simulink model "ExampleSimpleVehicle_PID"  (R2024b)
settings: Solver=ode1  StartTime=0.0  StopTime=inf  FixedStep=0.01  RelTol=1e-3
undefined symbols (not defined in the file or in its folder): DiscIntNeverNeededParam
libraries: rFproPhysicsLib x14, slpidlib x2, simulink x1
settings Model: ParamWorkspaceSource=ReferencedWorkspace  TunableVars=LOCAL_PORT_RECV,REMOTE_PORT_RECV,gCGHeight,gFrontTrack,gFrontWheelRadius,gLeftWheelBase,gRearTrack,gRearWheelRadius,gRightWheelBase  TunableVarsStorageClass=Auto,Auto,Auto,Auto,Auto,Auto,Auto,Auto,Auto  TunableVarsTypeQualifier=,,,,,,,,  Creator=enewton  LastModifiedBy=Saian
settings SolverCC: AlgebraicLoopSolver=TrustRegion
settings DataIOCC: LimitDataPoints=on  SaveFormat=Array  SignalLoggingSaveFormat=ModelDataLogs  SaveOutput=off  SignalLogging=off  DSMLogging=off  SaveTime=off  ReturnWorkspaceOutputs=off
settings OptimizationCC: BlockReduction=off  ConditionallyExecuteInputs=off  OptimizeBlockIOStorage=off  BufferReuse=off  GlobalBufferReuse=off  ExpressionFolding=off  ExpressionDepthLimit=2147483647  LocalBlockOutputs=off  LifeSpan=inf  OptimizeDataStoreBuffers=off  BusAssignmentInplaceUpdate=off
settings DebuggingCC: UnderspecifiedInitializationDetection=Classic  MergeDetectMultiDrivingBlocksExec=none  SolverPrmCheckMsg=warning  FcnCallInpInsideContextMsg=warning  UnconnectedInputMsg=warning  UnconnectedOutputMsg=warning  UnconnectedLineMsg=warning  StateNameClashWarn=warning  SFUnexpectedBacktrackingDiag=warning  SFNoUnconditionalDefaultTransitionDiag=warning  SFExecutionAtInitializationDiag=none  ArithmeticOperatorsInVariantConditions=warning
settings HardwareCC: ProdBitPerPointer=32  ProdBitPerSizeT=32  ProdBitPerPtrDiffT=32  ProdLargestAtomicFloat=None  ProdIntDivRoundTo=Undefined  ProdEndianess=Unspecified  ProdWordSize=32  ProdHWDeviceType=32-bit Generic
settings ModelReferenceCC: EnableRefExpFcnMdlSchedulingChecks=on  PropagateSignalLabelsOutOfModel=off
settings SFSimCC: SimUseLocalCustomCode=off  CustomCodeUndefinedFunction=UseInterfaceOnly  SimTargetLang=C++
settings RTWCC: Description=rFpro Target (Run Physics)  SystemTargetFile=rfpro.tlc  MakeCommand="make_rtw OPTS=\"-DRUN_PHYSICS\""  TemplateMakefile=rfpro.tmf  RTWUseLocalCustomCode=off  TargetLang=C++  GPUComputeCapability=3.5
settings CodeAppCC: StateflowObjectComments=on
settings STFCustomTargetCC: ModelReferenceCompliant=off  CombineOutputUpdateFcns=on  MatFileLogging=on  CPPClassGenCompliant=on  SystemTargetFile=rfpro.tlc
settings GRTTargetCC: TargetLangStandard=C89/C90 (ANSI)  ModelReferenceCompliant=off  ParMdlRefBuildCompliant=off  CompOptLevelCompliant=off  ConcurrentExecutionCompliant=off  UseToolchainInfoCompliant=off
settings ConfigComp: CovMetricSettings=dw  CovSaveCumulativeToWorkspaceVar=on  CovSaveSingleToWorkspaceVar=on  CovExternalEMLEnable=off

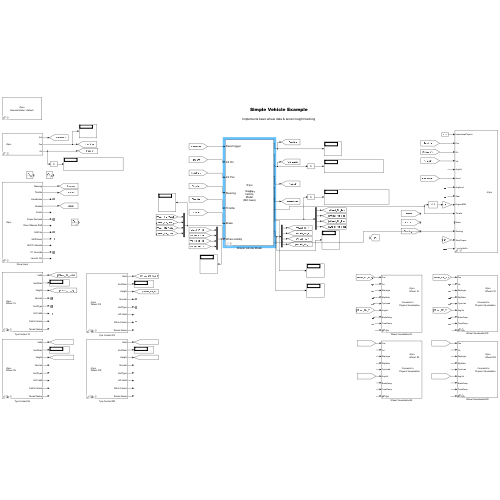
[thumbnail: Simulink's stored preview of the top-level diagram]
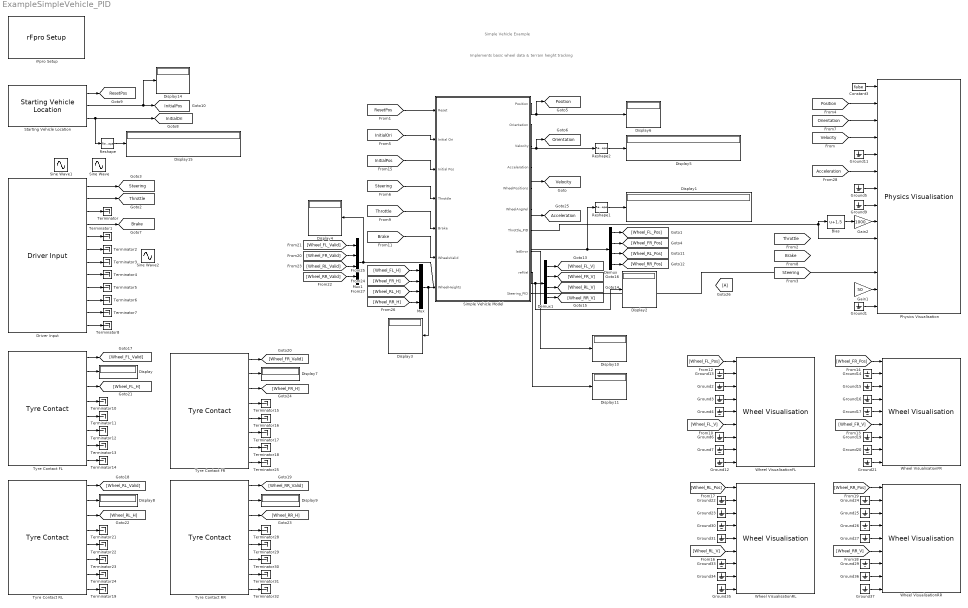
== system ExampleSimpleVehicle_PID ==
  note: Simple Vehicle Example
  note: Implements basic wheel data & terrain height tracking
  Bias : Bias  Bias=1.5  SaturateOnIntegerOverflow=off
  Constant3 : Constant  Value=false
  Demux : Demux
  Demux1 : Demux
  Display{,1..11,14..15} (14 alike) : Display
  "Driver Input " : rFproPhysicsLib/Driver Input
      settings: SourceProductName=rFpro Physics
  Gain1 : Gain  Gain=50
  Gain2 : Gain  Gain=1000
  Goto26 : Goto
  Ground{1..7,9,11..17,19..27,29..31,33..37} (32 alike) : Ground
  Mux : Mux
  Mux1 : Mux
  Physics Visualisation : rFproPhysicsLib/Physics Visualisation  PAR_SKIP_INTERNAL_PHYSICS=off  PAR_ACCEL_VALID=on  PAR_ROT_ACCEL_VALID=off  PAR_GEAR_VALID=off  PAR_RPM_VALID=on  PAR_INPUTS_VALID=on  PAR_STEER_TORQUE_VALID=on  PAR_HEADLIGHTS_ON_VALID=off  PAR_WHEEL_POS_VALID=on  PAR_WHEEL_ORI_VALID=off  PAR_TYRE_PARAMS_VALID=off  PAR_WHEEL_ROTATION_VALID=on  PAR_WHEEL_BRAKE_TEMP_VALID=off  PAR_WHEEL_TREAD_TEMP_VALID=off  PAR_WHEEL_AIR_TEMP_VALID=off  period=-1  offset=0  useReverseByteOrder=on  rFpro__platform=Remote Model - Default
      settings: SourceProductName=rFpro Physics
  Reshape : Reshape  OutputDimensionality=Customize  OutputDimensions=[3,3]
  Reshape1 : Reshape  OutputDimensionality=Customize  OutputDimensions=[3,4]
  Reshape2 : Reshape  OutputDimensionality=Customize  OutputDimensions=[3,3]
  Simple Vehicle Model : Subsystem  AncestorBlock=rFproPhysicsLib/Internal Utility/Simple Vehicle Model  mask(rFpro Simple Vehicle Model){TIMESTEP=0.01, gCGHeight=0.52, gLeftWheelBase=2.626, gRightWheelBase=2.626, gFrontTrack=1.55, gRearTrack=1.525, gFrontWheelRadius=0.32, gRearWheelRadius=0.33, gWheelDeflection=0}
      mask prompts: TIMESTEP "Sample time"; gCGHeight "Height of car body ref point"; gLeftWheelBase "Left Wheel Base"; gRightWheelBase "Right Wheel Base"; gFrontTrack "Front Wheel Track"; gRearTrack "Rear Wheel Track"; gFrontWheelRadius "Front wheel radius"; gRearWheelRadius "Rear wheel radius"; gWheelDeflection "Wheel Deflection"
      mask help:
      | Enter the car dimensions in metres.
      |
      | This block creates a CG_OFFSET_FROM_NOSE variable in the base workspace, for use by the "Starting Vehicle Location" block.
      mask init:
      | assignin('base', 'CG_OFFSET_FROM_NOSE', [-gLeftWheelBase/2, 0, gCGHeight]);
      mask DialogControl Container5 Prompt: Block Parameters
      mask DialogControl ParameterGroupVar Prompt: Vehicle Parameters
      mask Display:
      | disp('rFpro\n\nSimple\nVehicle\nModel\n(ISO Axes)')
      | port_label('input', 1, 'Reset trigger')
      | port_label('input', 2, 'Init Ori')
      | port_label('input', 3, 'Init Pos')
      | port_label('input', 4, 'Steering')
      | port_label('input', 5, 'Throttle')
      | port_label('input', 6, 'Brake')
      | port_label('input', 7, 'Wheel validity')
      | port_label('input', 8, 'Wheel heights')
      | 
      | port_label('output', 1, 'Position')
      | port_label('output', 2, 'Orientation')
      | port_label('output', 3, 'Velocity')
      | port_label('output', 4, 'Acceleration')
      | port_label('output', 5, 'Pos of Wheels')
      | port_label('output', 6, 'AngVel of Wheels')
  Sine Wave : Sin  SampleTime=0
  Sine Wave1 : Sin  Amplitude=0.5  Bias=0.5  Phase=pi  SampleTime=0
  Sine Wave2 : Sin  Amplitude=0.5  Bias=0.5  SampleTime=0
  Starting Vehicle Location : rFproPhysicsLib/Starting Vehicle Location  cg_offset=CG_OFFSET_FROM_NOSE  numPackets=1  rFpro__platform=Remote Model - Default
      settings: SourceProductName=rFpro Physics
  Terminator{,1..8,10..19,21..25,28..32} (29 alike) : Terminator
  Tyre Contact FL : rFproPhysicsLib/Tyre Contact  LabelModeActiveChoice=rFproLib_RemoteModel  wheel=FL  contact=[]  radius=0.3  width=0.32  sampleTime=0.001  rFpro__platform=Remote Model - Default
      settings: SourceProductName=rFpro Physics
  Tyre Contact FR : rFproPhysicsLib/Tyre Contact  LabelModeActiveChoice=rFproLib_RemoteModel  wheel=FR  contact=[]  radius=0.32  width=0.25  sampleTime=0.001  rFpro__platform=Remote Model - Default
      settings: SourceProductName=rFpro Physics
  Tyre Contact RL : rFproPhysicsLib/Tyre Contact  LabelModeActiveChoice=rFproLib_RemoteModel  wheel=RL  contact=[]  radius=0.33  width=0.25  sampleTime=0.001  rFpro__platform=Remote Model - Default
      settings: SourceProductName=rFpro Physics
  Tyre Contact RR : rFproPhysicsLib/Tyre Contact  LabelModeActiveChoice=rFproLib_RemoteModel  wheel=RR  contact=[]  radius=0.33  width=0.25  sampleTime=0.001  rFpro__platform=Remote Model - Default
      settings: SourceProductName=rFpro Physics
  Wheel VisualisationFL : rFproPhysicsLib/Wheel Visualisation  wheelStr=FL
      settings: SourceProductName=rFpro Physics
  Wheel VisualisationFR : rFproPhysicsLib/Wheel Visualisation  wheelStr=FR
      settings: SourceProductName=rFpro Physics
  Wheel VisualisationRL : rFproPhysicsLib/Wheel Visualisation  wheelStr=RL
      settings: SourceProductName=rFpro Physics
  Wheel VisualisationRR : rFproPhysicsLib/Wheel Visualisation  wheelStr=RR
      settings: SourceProductName=rFpro Physics
  rFpro Setup : rFproPhysicsLib/rFpro Setup  platform=Remote Model - Default  stopOnSessionEnd=on  usePseudoRealtime=on  syncToRF=on  useReverseByteOrder=off  useRfTime=on  minIterations=4  maxIterations=1000  ipReceiveAddress='127.0.0.1'  ipReceivePort=11054  receiveSampleTime=-1  ipTransmitAddress='127.0.0.1'  ipTransmitPort=11052  transmitSampleTime=-1  pluginType=RUN_PHYSICS  sysTarget=xpctarget.tlc  templateMakeFile=xpc_default_tmf  makeCommand=make_rtw  buildDesc=xPC target
      settings: SourceProductName=rFpro Physics
  tag scope: Acceleration=global, Brake=global, InitialOri=global, InitialPos=global, Orientation=global, Position=global, ResetPos=global, Steering=global, Throttle=global, Velocity=global
  wires:
  Starting Vehicle Location/2 -> Display14/1, [InitialPos]
  Constant3/1 -> Physics Visualisation/1
  [Orientation] -> Physics Visualisation/3
  [Velocity] -> Physics Visualisation/4
  [Position] -> Physics Visualisation/2
  "Driver Input "/3 -> Terminator/1
  "Driver Input "/5 -> Terminator1/1
  "Driver Input "/6 -> Terminator2/1
  "Driver Input "/7 -> Terminator3/1
  "Driver Input "/8 -> Terminator4/1
  "Driver Input "/9 -> Terminator5/1
  "Driver Input "/10 -> Terminator6/1
  "Driver Input "/11 -> Terminator7/1
  "Driver Input "/12 -> Terminator8/1
  [Acceleration] -> Physics Visualisation/6
  Ground9/1 -> Physics Visualisation/8
  Gain2/1 -> Physics Visualisation/9
  Ground11/1 -> Physics Visualisation/5
  Starting Vehicle Location/1 -> [ResetPos]
  Gain1/1 -> Physics Visualisation/13
  Ground1/1 -> Physics Visualisation/14
  Tyre Contact FL/4 -> Terminator10/1
  Tyre Contact FL/5 -> Terminator11/1
  Tyre Contact FL/6 -> Terminator12/1
  Ground2/1 -> Wheel VisualisationFL/3
  Ground3/1 -> Wheel VisualisationFL/4
  Ground4/1 -> Wheel VisualisationFL/5
  Ground6/1 -> Wheel VisualisationFL/7
  Ground7/1 -> Wheel VisualisationFL/8
  Ground12/1 -> Wheel VisualisationFL/9
  Ground13/1 -> Wheel VisualisationFL/2
  Tyre Contact FL/7 -> Terminator13/1
  Tyre Contact FL/2 -> Display/1
  Tyre Contact FL/8 -> Terminator14/1
  Tyre Contact FR/5 -> Terminator16/1
  Tyre Contact FR/6 -> Terminator17/1
  Tyre Contact FR/7 -> Terminator18/1
  Tyre Contact FR/2 -> Display7/1
  Tyre Contact RL/4 -> Terminator21/1
  Tyre Contact RL/5 -> Terminator22/1
  Tyre Contact RL/6 -> Terminator23/1
  Tyre Contact RL/7 -> Terminator24/1
  Tyre Contact RL/2 -> Display8/1
  Tyre Contact RL/8 -> Terminator19/1
  Tyre Contact RR/5 -> Terminator29/1
  Tyre Contact RR/6 -> Terminator30/1
  Tyre Contact RR/7 -> Terminator31/1
  Tyre Contact RR/2 -> Display9/1
  Ground14/1 -> Wheel VisualisationFR/2
  Ground15/1 -> Wheel VisualisationFR/3
  Ground16/1 -> Wheel VisualisationFR/4
  Ground17/1 -> Wheel VisualisationFR/5
  Ground19/1 -> Wheel VisualisationFR/7
  Ground20/1 -> Wheel VisualisationFR/8
  Ground21/1 -> Wheel VisualisationFR/9
  Ground22/1 -> Wheel VisualisationRL/2
  Ground23/1 -> Wheel VisualisationRL/3
  Ground30/1 -> Wheel VisualisationRL/4
  Ground31/1 -> Wheel VisualisationRL/5
  Ground33/1 -> Wheel VisualisationRL/7
  Ground34/1 -> Wheel VisualisationRL/8
  Ground35/1 -> Wheel VisualisationRL/9
  Ground24/1 -> Wheel VisualisationRR/2
  Ground25/1 -> Wheel VisualisationRR/3
  Ground26/1 -> Wheel VisualisationRR/4
  Ground27/1 -> Wheel VisualisationRR/5
  Ground29/1 -> Wheel VisualisationRR/7
  Ground36/1 -> Wheel VisualisationRR/8
  Ground37/1 -> Wheel VisualisationRR/9
  Ground5/1 -> Physics Visualisation/7
  Starting Vehicle Location/3 -> Reshape/1, [InitialOri]
  [InitialOri] -> Simple Vehicle Model/2(Initial Ori)
  [ResetPos] -> Simple Vehicle Model/1(Reset)
  [Throttle] -> Simple Vehicle Model/5(Brake)
  [Brake] -> Simple Vehicle Model/6(WheelsValid)
  [InitialPos] -> Simple Vehicle Model/3(Initial Pos)
  [Steering] -> Simple Vehicle Model/4(Throttle)
  Simple Vehicle Model/5(WheelPositions) -> Reshape1/1, Demux/1
  Tyre Contact FR/4 -> Terminator15/1
  Tyre Contact FR/8 -> Terminator25/1
  Simple Vehicle Model/1(Position) -> Display6/1, [Position]
  Simple Vehicle Model/2(Orientation) -> [Orientation], Reshape2/1
  Simple Vehicle Model/3(Velocity) -> [Velocity]
  Demux/1 -> [Wheel_FL_Pos]
  Demux/2 -> [Wheel_FR_Pos]
  Demux/3 -> [Wheel_RL_Pos]
  Demux/4 -> [Wheel_RR_Pos]
  Demux1/1 -> [Wheel_FL_V]
  Demux1/2 -> [Wheel_FR_V]
  Demux1/3 -> [Wheel_RL_V]
  Demux1/4 -> [Wheel_RR_V]
  Simple Vehicle Model/6(WheelAngVel) -> Display2/1, Demux1/1
  [Wheel_FL_Pos] -> Wheel VisualisationFL/1
  [Wheel_FL_V] -> Wheel VisualisationFL/6
  [Wheel_FR_Pos] -> Wheel VisualisationFR/1
  [Wheel_FR_V] -> Wheel VisualisationFR/6
  [Wheel_RL_V] -> Wheel VisualisationRL/6
  [Wheel_RL_Pos] -> Wheel VisualisationRL/1
  [Wheel_RR_V] -> Wheel VisualisationRR/6
  [Wheel_RR_Pos] -> Wheel VisualisationRR/1
  Tyre Contact RL/1 -> [Wheel_RL_Valid]
  Tyre Contact RL/3 -> [Wheel_RL_H]
  Tyre Contact RR/1 -> [Wheel_RR_Valid]
  Tyre Contact RR/3 -> [Wheel_RR_H]
  Tyre Contact FR/3 -> [Wheel_FR_H]
  Tyre Contact FR/1 -> [Wheel_FR_Valid]
  Tyre Contact FL/1 -> [Wheel_FL_Valid]
  Tyre Contact FL/3 -> [Wheel_FL_H]
  [Wheel_RL_Valid] -> Mux1/3
  [Wheel_RR_Valid] -> Mux1/4
  [Wheel_FL_Valid] -> Mux1/1
  [Wheel_FR_Valid] -> Mux1/2
  [Wheel_FR_H] -> Mux/2
  [Wheel_FL_H] -> Mux/1
  [Wheel_RR_H] -> Mux/4
  [Wheel_RL_H] -> Mux/3
  Mux1/1 -> Display4/1, Simple Vehicle Model/7(WheelHeights)
  Mux/1 -> Display3/1
  Tyre Contact RR/4 -> Terminator28/1
  Tyre Contact RR/8 -> Terminator32/1
  Reshape/1 -> Display15/1
  Reshape1/1 -> Display1/1
  Reshape2/1 -> Display5/1
  Bias/1 -> Gain2/1
  Simple Vehicle Model/4(Acceleration) -> [Acceleration]
  "Driver Input "/1 -> [Steering]
  "Driver Input "/2 -> [Throttle]
  "Driver Input "/4 -> [Brake]
  Simple Vehicle Model/8(latError) -> Display10/1
  Simple Vehicle Model/9(refVel) -> Display11/1
  Simple Vehicle Model/7(Throttle_PID) -> Bias/1, Physics Visualisation/10
  Simple Vehicle Model/10(Steering_PID) -> Physics Visualisation/12

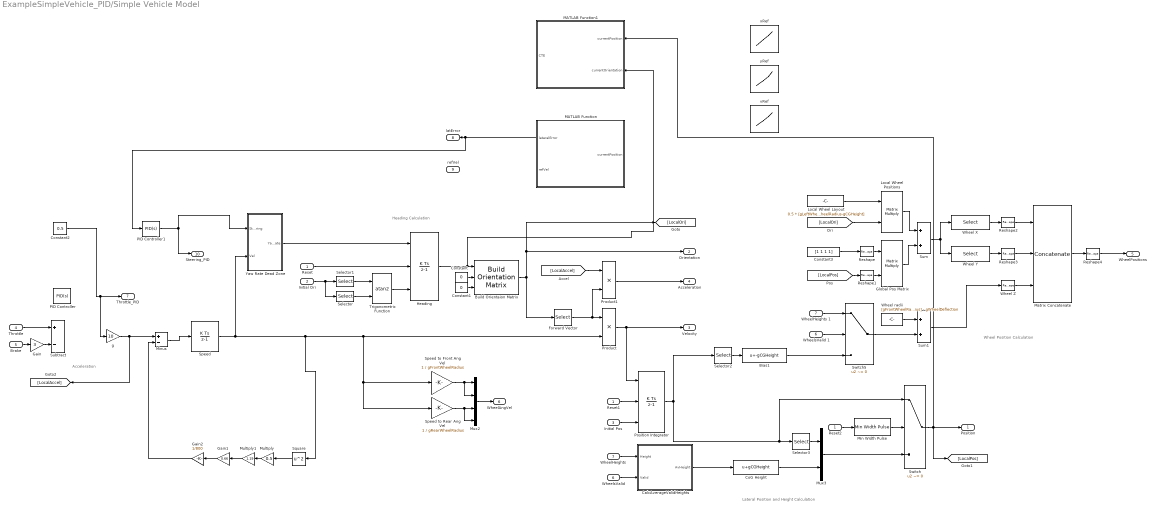
== system ExampleSimpleVehicle_PID/Simple Vehicle Model ==
  note: Wheel Position Calculation
  note: Acceleration
  note: Heading Calculation
  note: Lateral Position and Height Calculation
  Reset : Inport
  Initial Ori : Inport  Port=2
  Initial Pos : Inport  Port=3
  Throttle : Inport  Port=4
  Brake : Inport  Port=5
  WheelsValid : Inport  Port=6
  WheelHeights : Inport  Port=7
  Bias1 : Bias  Bias=-gCGHeight  SaturateOnIntegerOverflow=off
  Build Orientaion Matrix : rFproPhysicsLib/Build Orientation Matrix  ISOAxes=on  YPROrder=on
      settings: SourceProductName=rFpro Physics
  CalcAverageValidHeights : Subsystem
  CoG Height : Bias  Bias=gCGHeight  SaturateOnIntegerOverflow=off
  Constant : Constant  Value=0
  Constant1 : Constant  Value=0
  Constant2 : Constant  Value=0.5
  Constant3 : Constant  Value=[1 1 1 1]
  Forward Vector : Selector  NumberOfDimensions=2  InputPortWidth=3  IndexOptions=Index vector (dialog),Index vector (dialog)  Indices=1,1:3  OutputSizes=1,1
  Gain : Gain  Gain=3
  Gain1 : Gain  Gain=0.66
  Gain2 : Gain  Gain=1/800
  Global Pos Matrix : Product  Multiplication=Matrix(*)
  Heading : DiscreteIntegrator  ExternalReset=level  InitialConditionSource=external  SampleTime=TIMESTEP  ICPrevOutput=DiscIntNeverNeededParam  ICPrevScaledInput=DiscIntNeverNeededParam
  Local Wheel Positions : Product  Multiplication=Matrix(*)  RndMeth=Zero
  Local Wheel Layout : Constant  Value="0.5 * [gLeftWheelBase,   gFrontTrack, gFrontWheelRadius-gCGHeight; gRightWheelBase, -gFrontTrack, gFrontWheelRadius-gCGHeight; -gLeftWheelBase,   gRearTrack,  gRearWheelRadius-gCGHeight; -gRightWheelBase, -gRearTrack,  gRearWheelRadius-gCGHeight]"
  MATLAB Function : MATLAB Function  TreatAsAtomicUnit=on
  MATLAB Function1 : MATLAB Function  AncestorBlock=rFproPhysicsLib/Internal Utility/Simple Vehicle Model/MATLAB Function  TreatAsAtomicUnit=on
  Matrix Concatenate : Concatenate  NumInputs=3  Mode=Multidimensional array
  Min Width Pulse : rFproPhysicsLib/Internal Utility/Min Width Pulse  width=20
      settings: SourceProductName=rFpro Physics
  Minus : Sum  Inputs=+-
  Multiply : Gain  Gain=0.5
  Multiply1 : Gain  Gain=1.19
  Mux2 : Mux
  Mux3 : Mux  Inputs=2
  PID Controller : slpidlib/PID Controller  Controller=PID  Form=Parallel  TimeDomain=Continuous-time  UseExternalTs=off  SampleTime=-1  IntegratorMethod=Forward Euler  FilterMethod=Forward Euler  ControllerParametersSource=internal  P=1  I=0  UseKiTs=off  D=5  UseExternalDerivativeSource=off  N=100  UseFilter=on  TunerSelectOption=Transfer Function Based (PID Tuner App)  InitialConditionSource=internal  InitialConditionForIntegrator=0  InitialConditionForFilter=0  DifferentiatorICPrevScaledInput=0  ExternalReset=none  TrackingMode=off  Kt=1  LimitOutput=on  SatLimitsSource=internal  UpperSaturationLimit=1  LowerSaturationLimit=-1  LinearizeAsGain=on  AntiWindupMode=none  Kb=1  LimitIntegrator=off  UpperIntegratorSaturationLimit=inf  LowerIntegratorSaturationLimit=-inf  POutMin=[]  POutMax=[]  IOutMin=[]  IOutMax=[]  DOutMin=[]  DOutMax=[]  NOutMin=[]  NOutMax=[]  SumOutMin=[]  SumOutMax=[]  SaturationOutMin=[]  SaturationOutMax=[]  PParamMin=[]  PParamMax=[]  IParamMin=[]  IParamMax=[]  DParamMin=[]  DParamMax=[]  NParamMin=[]  NParamMax=[]  KbParamMin=[]  KbParamMax=[]  KtParamMin=[]  KtParamMax=[]  KbOutMin=[]  KbOutMax=[]  KtOutMin=[]  KtOutMax=[]  IntegratorOutMin=[]  IntegratorOutMax=[]  FilterOutMin=[]  FilterOutMax=[]  SumI1OutMin=[]  SumI1OutMax=[]  SumI2OutMin=[]  SumI2OutMax=[]  SumI3OutMin=[]  SumI3OutMax=[]  SumI4OutMin=[]  SumI4OutMax=[]  SumDOutMin=[]  SumDOutMax=[]  DifferentiatorOutMin=[]  DifferentiatorOutMax=[]  FilterDiffOutCoefMin=[]  FilterDiffOutCoefMax=[]  ReciprocalOutMin=[]  ReciprocalOutMax=[]  SumDenOutMin=[]  SumDenOutMax=[]  SumNumOutMin=[]  SumNumOutMax=[]  DivideOutMin=[]  DivideOutMax=[]  UdiffTsProdOutMin=[]  UdiffTsProdOutMax=[]  NTsProdOutMin=[]  NTsProdOutMax=[]  UintegralTsProdOutMin=[]  UintegralTsProdOutMax=[]  UngainTsProdOutMin=[]  UngainTsProdOutMax=[]  ClampingZeroOutDataTypeStr=Inherit: Inherit via back propagation  ClampingZeroOutMin=[]  ClampingZeroOutMax=[]  FilterDenConstantOutDataTypeStr=Inherit: Inherit via back propagation  FilterDenConstantOutMin=[]  FilterDenConstantOutMax=[]  PCopyOutDataTypeStr=Inherit: Inherit via back propagation  PCopyOutMin=[]  PCopyOutMax=[]  NCopyOutDataTypeStr=Inherit: Inherit via back propagation  NCopyOutMin=[]  NCopyOutMax=[]  IntegratorContinuousStateAttributes=''  IntegratorStateMustResolveToSignalObject=off  IntegratorRTWStateStorageClass=Auto  FilterContinuousStateAttributes=''  FilterStateMustResolveToSignalObject=off  FilterRTWStateStorageClass=Auto  ParallelPVariant=InternalParameters  IdealPVariant=Disabled  IVariant=InternalParameters  DVariant=InternalParameters  IntegratorVariant=Continuous  SatVariant=Enabled  AWVariant=Passthrough  PCopyVariant=Disabled  TRVariant=Disabled  FdbkBlocksVariant=Forward  IdealPFdbkVariant=Disabled  SatFdbkVariant=Disabled  DerivativeFilterVariant=ContFilter  NVariant=InternalParameters  NCopyVariant=Disabled  FilterICVariant=InternalICsFilter  IntegratorICVariant=InternalICs  ExternalResetVariant=Disabled  TRSumVariant=Passthrough  SumFdbkVariant=Disabled  SumVariant=Sum_PID  TsampFilterVariant=InternalTs  TsampNgainVariant=Passthrough  TsampIntegralVariant=Disabled_SignalSpec  ExternalSaturationOutDataTypeStr=Inherit: Same as second input  DerivativeSourceVariant=ErrorSignal  PreIntVariant=InternalPreInt
  PID Controller1 : slpidlib/PID Controller  Controller=PID  Form=Parallel  TimeDomain=Continuous-time  UseExternalTs=off  SampleTime=-1  IntegratorMethod=Forward Euler  FilterMethod=Forward Euler  ControllerParametersSource=internal  P=1  I=0  UseKiTs=off  D=5  UseExternalDerivativeSource=off  N=100  UseFilter=on  TunerSelectOption=Transfer Function Based (PID Tuner App)  InitialConditionSource=internal  InitialConditionForIntegrator=0  InitialConditionForFilter=0  DifferentiatorICPrevScaledInput=0  ExternalReset=none  TrackingMode=off  Kt=1  LimitOutput=on  SatLimitsSource=internal  UpperSaturationLimit=1  LowerSaturationLimit=-1  LinearizeAsGain=on  AntiWindupMode=none  Kb=1  LimitIntegrator=off  UpperIntegratorSaturationLimit=inf  LowerIntegratorSaturationLimit=-inf  POutMin=[]  POutMax=[]  IOutMin=[]  IOutMax=[]  DOutMin=[]  DOutMax=[]  NOutMin=[]  NOutMax=[]  SumOutMin=[]  SumOutMax=[]  SaturationOutMin=[]  SaturationOutMax=[]  PParamMin=[]  PParamMax=[]  IParamMin=[]  IParamMax=[]  DParamMin=[]  DParamMax=[]  NParamMin=[]  NParamMax=[]  KbParamMin=[]  KbParamMax=[]  KtParamMin=[]  KtParamMax=[]  KbOutMin=[]  KbOutMax=[]  KtOutMin=[]  KtOutMax=[]  IntegratorOutMin=[]  IntegratorOutMax=[]  FilterOutMin=[]  FilterOutMax=[]  SumI1OutMin=[]  SumI1OutMax=[]  SumI2OutMin=[]  SumI2OutMax=[]  SumI3OutMin=[]  SumI3OutMax=[]  SumI4OutMin=[]  SumI4OutMax=[]  SumDOutMin=[]  SumDOutMax=[]  DifferentiatorOutMin=[]  DifferentiatorOutMax=[]  FilterDiffOutCoefMin=[]  FilterDiffOutCoefMax=[]  ReciprocalOutMin=[]  ReciprocalOutMax=[]  SumDenOutMin=[]  SumDenOutMax=[]  SumNumOutMin=[]  SumNumOutMax=[]  DivideOutMin=[]  DivideOutMax=[]  UdiffTsProdOutMin=[]  UdiffTsProdOutMax=[]  NTsProdOutMin=[]  NTsProdOutMax=[]  UintegralTsProdOutMin=[]  UintegralTsProdOutMax=[]  UngainTsProdOutMin=[]  UngainTsProdOutMax=[]  ClampingZeroOutDataTypeStr=Inherit: Inherit via back propagation  ClampingZeroOutMin=[]  ClampingZeroOutMax=[]  FilterDenConstantOutDataTypeStr=Inherit: Inherit via back propagation  FilterDenConstantOutMin=[]  FilterDenConstantOutMax=[]  PCopyOutDataTypeStr=Inherit: Inherit via back propagation  PCopyOutMin=[]  PCopyOutMax=[]  NCopyOutDataTypeStr=Inherit: Inherit via back propagation  NCopyOutMin=[]  NCopyOutMax=[]  IntegratorContinuousStateAttributes=''  IntegratorStateMustResolveToSignalObject=off  IntegratorRTWStateStorageClass=Auto  FilterContinuousStateAttributes=''  FilterStateMustResolveToSignalObject=off  FilterRTWStateStorageClass=Auto  ParallelPVariant=InternalParameters  IdealPVariant=Disabled  IVariant=InternalParameters  DVariant=InternalParameters  IntegratorVariant=Continuous  SatVariant=Enabled  AWVariant=Passthrough  PCopyVariant=Disabled  TRVariant=Disabled  FdbkBlocksVariant=Forward  IdealPFdbkVariant=Disabled  SatFdbkVariant=Disabled  DerivativeFilterVariant=ContFilter  NVariant=InternalParameters  NCopyVariant=Disabled  FilterICVariant=InternalICsFilter  IntegratorICVariant=InternalICs  ExternalResetVariant=Disabled  TRSumVariant=Passthrough  SumFdbkVariant=Disabled  SumVariant=Sum_PID  TsampFilterVariant=InternalTs  TsampNgainVariant=Passthrough  TsampIntegralVariant=Disabled_SignalSpec  ExternalSaturationOutDataTypeStr=Inherit: Same as second input  DerivativeSourceVariant=ErrorSignal  PreIntVariant=InternalPreInt
  Position Integrator : DiscreteIntegrator  ExternalReset=level  InitialConditionSource=external  SampleTime=TIMESTEP  ICPrevOutput=DiscIntNeverNeededParam  ICPrevScaledInput=DiscIntNeverNeededParam
  Product : Product  RndMeth=Zero
  Product1 : Product  RndMeth=Zero
  Reset1 : InportShadow
  Reset2 : InportShadow
  Reshape : Reshape  OutputDimensionality=Column vector (2-D)
  Reshape1 : Reshape  OutputDimensionality=Row vector (2-D)
  Reshape2 : Reshape  OutputDimensionality=Row vector (2-D)
  Reshape3 : Reshape  OutputDimensionality=Row vector (2-D)
  Reshape4 : Reshape
  Selector : Selector  NumberOfDimensions=2  InputPortWidth=3  IndexOptions=Index vector (dialog),Index vector (dialog)  Indices=1,1  OutputSizes=1,1
  Selector1 : Selector  NumberOfDimensions=2  InputPortWidth=3  IndexOptions=Index vector (dialog),Index vector (dialog)  Indices=1,2  OutputSizes=1,1
  Selector2 : Selector  InputPortWidth=3  IndexOptions=Index vector (dialog)  Indices=3  OutputSizes=1
  Selector3 : Selector  InputPortWidth=3  IndexOptions=Index vector (dialog)  Indices=[1 2]  OutputSizes=1
  Speed : DiscreteIntegrator  SampleTime=TIMESTEP  LimitOutput=on  LowerSaturationLimit=0  ICPrevOutput=DiscIntNeverNeededParam  ICPrevScaledInput=DiscIntNeverNeededParam
  Speed to Front Ang Vel : Gain  Gain=1 / gFrontWheelRadius
  Speed to Rear Ang Vel : Gain  Gain=1 / gRearWheelRadius
  Square : Math  Operator=square
  Subtract : Sum  Inputs=+-
  Sum : Sum
  Sum1 : Sum
  Switch : Switch  Criteria=u2 ~= 0  SaturateOnIntegerOverflow=off  InputSameDT=off
  Switch5 : Switch  Criteria=u2 ~= 0  SaturateOnIntegerOverflow=off  InputSameDT=off
  Trigonometric Function : Trigonometry  Operator=atan2
  Wheel X : Selector  NumberOfDimensions=2  InputPortWidth=3  IndexOptions=Select all,Index vector (dialog)  Indices=[1 3],1  OutputSizes=1,1
  Wheel Y : Selector  NumberOfDimensions=2  InputPortWidth=3  IndexOptions=Select all,Index vector (dialog)  Indices=[1 3],2  OutputSizes=1,1
  Wheel Z : Reshape  OutputDimensionality=Row vector (2-D)
  Wheel radii : Constant  Value=[gFrontWheelRadius, gFrontWheelRadius, gRearWheelRadius, gRearWheelRadius] - gWheelDeflection
  WheelHeights 1 : InportShadow  Port=7
  WheelsValid 1 : InportShadow  Port=6
  Yaw Rate Dead Zone : Subsystem
  g : Gain  Gain=10
  vRef : Lookup_n-D  NumberOfTableDimensions=1  BreakpointsForDimension1=[1 2 3 4 5 6 7 8 9 10 11 12 13 14 15 16 17 18 19 20 21 22 23 24 25 26 27 28 29 30 31 32 33 34 35 36 37 38 39 40 41 42 43 44 45 46 47 48 49 50 51 52 53 54 55 56 57 58 59 60 61 62 63 64 65 66 67 68 69 70 71 72 73 74 75 76 77 78 79 80 81 82 83 84 85 86 87 88 89 90 91 92 93 94 95 96 97 98 99 100 101 102 103 104 105 106 107 108 109 110 111 112 113 114 115 116 117 118 119 120 121 122 123 124 125 126 127 128 129 130 131 132 133 134 135 136 137 138 139 140 141 142 143 144 145]  Table=[70;66.2941526152573;65.4883647028928;66.0806810173367;65.26896339678061;66.38411146223039;67.3958387030261;67.44592545744069;69.329950287306;69.1882758068728;68.3399139325445;67.8708656511444;68.0298306929415;68.5896149793253;68.1152248297563;68.63555972456859;69.1481986236618;69.4599993837293;69.9252960878933;69.3639988911179;69.8107068477354;69.8743668318338;69.619725001083;69.7562053585058;69.5126574618636;66.8719643020907;66.5091815156028;63.7827888901593;61.4788133988011;57.7449016550197;53.9974942907394;53.6605244902812;52.084372378414;50.7040292465574;48.3551543600423;47.8757137938598;45.44230021571;45.0547902412987;44.8125277874768;44.1542423154531;42.7562947109367;43.0237595384218;42.9484526008551;41.4257959721631;43.2571984505023;43.5174230788054;42.7218682523597;42.8210740638573;43.8798605976025;43.3680625384228;41.050532484812;41.1167068038216;41.5115895718732;40.9821406887103;40.9724706479303;40.3572685751828;39.8779433001052;40.8523153006594;43.4782648280148;46.1514165633422;51.1173397417285;59.1586834051362;63.8222944745662;64.9860662503273;68.09774394366831;63.3540045110797;62.8833170176386;63.6684950949253;61.9666887077676;62.2677836847414;63.582020518799;63.7412538286618;67.1728885787014;69.1240638051038;68.2678328545159;66.2320071591884;64.9379557107406;66.9499315721812;68.288600479504;68.7439476332636;69.3231332765677;69.8500899327105;68.66563066099511;69.50160418981601;69.596479219993;69.6746981329475;69.8776836020929;69.8129239020713;69.9633846068996;69.8356926516352;69.9605815921807;69.99484195273639;69.76728865106691;69.8972515280409;69.946697957835;69.8660412195262;69.8644375826603;69.5234982627379;64.634943151824;68.6108023038381;63.4034940082739;61.3828028681508;59.1949084097623;56.0993056497234;52.9563000761606;48.6600632149421;46.5811102623243;45.3740766116321;44.0924658888451;43.4590924152461;42.1678712337758;43.2439583256756;43.5724926564217;43.4993836022364;43.2285780638725;43.4716042905227;48.3773165515135;42.6594142234564;41.4769704966752;41.490023311183;40.1153820764336;39.439060283349;40.7167392521961;41.7807093964386;44.0168794632518;47.2964084120581;49.8703327366803;54.2578101978239;48.7811919622444;48.888182493106;47.7142112915798;46.8807887059169;46.4014281715362;46.2575661895888;46.9478486843666;50.2626308688873;50.659172156746;53.7892565325441;55.7629716999758;62.0428321692388;65.39425033502739;61.3094080047088;66.1398697765437;55.8306766985528;70]  InternalRulePriority=Speed  RndMeth=Simplest
  xRef : Lookup_n-D  NumberOfTableDimensions=1  BreakpointsForDimension1=[1:145]  Table=[-293.551;-288.888;-284.234;-279.706;-275.116;-270.658;-266.15;-261.572;-257.07;-252.512;-248.118;-243.621;-238.948;-234.252;-229.748;-225.108;-220.448;-215.821;-211.368;-206.689;-202.019;-197.514;-192.734;-188.173;-183.409;-178.862;-174.111;-169.518;-165.028;-160.426;-155.615;-150.805;-145.972;-141.051;-136.113;-131.172;-126.225;-121.479;-116.839;-112.231;-107.63;-103.293;-99.172;-95.29000000000001;-91.904;-88.824;-86.108;-83.89400000000001;-82.10899999999999;-80.684;-79.68300000000001;-79.193;-79.18300000000001;-79.658;-80.649;-82.20099999999999;-84.31699999999999;-86.785;-89.604;-92.767;-96.381;-100.164;-103.811;-107.724;-111.675;-115.986;-120.236;-124.445;-128.896;-133.178;-137.479;-142.074;-146.662;-151.29;-155.903;-160.379;-165.098;-169.788;-174.364;-179.038;-183.745;-188.228;-192.718;-197.269;-202.011;-206.683;-211.409;-216.257;-221.024;-225.706;-230.57;-235.133;-239.716;-244.441;-249.136;-254.059;-258.81;-263.396;-267.885;-272.623;-277.325;-282.002;-286.667;-291.335;-296.087;-300.986;-305.893;-310.844;-315.998;-321.066;-326.146;-330.974;-335.709;-340.226;-344.401;-348.189;-351.562;-354.727;-357.385;-359.545;-361.269;-362.446;-363.009;-362.989;-362.43;-361.461;-360.141;-358.422;-356.517;-354.364;-351.832;-348.878;-345.485;-341.805;-337.808;-333.74;-329.372;-324.962;-320.24;-315.421;-310.547;-305.622;-300.983;-295.871;-293.551]  InternalRulePriority=Speed  RndMeth=Simplest
  yRef : Lookup_n-D  NumberOfTableDimensions=1  BreakpointsForDimension1=[1:145]  Table=[-293.551;-288.888;-284.234;-279.706;-275.116;-270.658;-266.15;-261.572;-257.07;-252.512;-248.118;-243.621;-238.948;-234.252;-229.748;-225.108;-220.448;-215.821;-211.368;-206.689;-202.019;-197.514;-192.734;-188.173;-183.409;-178.862;-174.111;-169.518;-165.028;-160.426;-155.615;-150.805;-145.972;-141.051;-136.113;-131.172;-126.225;-121.479;-116.839;-112.231;-107.63;-103.293;-99.172;-95.29000000000001;-91.904;-88.824;-86.108;-83.89400000000001;-82.10899999999999;-80.684;-79.68300000000001;-79.193;-79.18300000000001;-79.658;-80.649;-82.20099999999999;-84.31699999999999;-86.785;-89.604;-92.767;-96.381;-100.164;-103.811;-107.724;-111.675;-115.986;-120.236;-124.445;-128.896;-133.178;-137.479;-142.074;-146.662;-151.29;-155.903;-160.379;-165.098;-169.788;-174.364;-179.038;-183.745;-188.228;-192.718;-197.269;-202.011;-206.683;-211.409;-216.257;-221.024;-225.706;-230.57;-235.133;-239.716;-244.441;-249.136;-254.059;-258.81;-263.396;-267.885;-272.623;-277.325;-282.002;-286.667;-291.335;-296.087;-300.986;-305.893;-310.844;-315.998;-321.066;-326.146;-330.974;-335.709;-340.226;-344.401;-348.189;-351.562;-354.727;-357.385;-359.545;-361.269;-362.446;-363.009;-362.989;-362.43;-361.461;-360.141;-358.422;-356.517;-354.364;-351.832;-348.878;-345.485;-341.805;-337.808;-333.74;-329.372;-324.962;-320.24;-315.421;-310.547;-305.622;-300.983;-295.871;-293.551]  InternalRulePriority=Speed  RndMeth=Simplest
  Position : Outport  VectorParamsAs1DForOutWhenUnconnected=off
  Orientation : Outport  Port=2  VectorParamsAs1DForOutWhenUnconnected=off
  Velocity : Outport  Port=3  VectorParamsAs1DForOutWhenUnconnected=off
  Acceleration : Outport  Port=4  VectorParamsAs1DForOutWhenUnconnected=off
  WheelPositions : Outport  Port=5  VectorParamsAs1DForOutWhenUnconnected=off
  WheelAngVel : Outport  Port=6  VectorParamsAs1DForOutWhenUnconnected=off
  Throttle_PID : Outport  Port=7
  latError : Outport  Port=8
  refVel : Outport  Port=9
  Steering_PID : Outport  Port=10
  wires:
  PID Controller1/1 -> Yaw Rate Dead Zone/1(Steering), Steering_PID/1
  Throttle/1 -> Subtract/1
  Minus/1 -> Speed/1
  Gain2/1 -> Minus/2
  Gain1/1 -> Gain2/1
  Multiply/1 -> Multiply1/1
  Square/1 -> Multiply/1
  Multiply1/1 -> Gain1/1
  Product1/1 -> Acceleration/1
  [LocalAccel] -> Product1/1
  Speed to Rear Ang Vel/1 -> Mux2/3, Mux2/4
  Reshape4/1 -> WheelPositions/1
  Matrix Concatenate/1 -> Reshape4/1
  Wheel Z/1 -> Matrix Concatenate/3
  Reshape3/1 -> Matrix Concatenate/2
  Wheel Y/1 -> Reshape3/1
  Reshape2/1 -> Matrix Concatenate/1
  Wheel X/1 -> Reshape2/1
  Sum1/1 -> Wheel Z/1
  Wheel radii/1 -> Sum1/1
  Sum/1 -> Wheel X/1, Wheel Y/1
  WheelHeights 1/1 -> Switch5/1
  WheelsValid 1/1 -> Switch5/2
  Switch5/1 -> Sum1/2
  Global Pos Matrix/1 -> Sum/2
  Local Wheel Positions/1 -> Sum/1
  [LocalOri] -> Local Wheel Positions/2
  Reshape1/1 -> Global Pos Matrix/2
  Reshape/1 -> Global Pos Matrix/1
  [LocalPos] -> Reshape1/1
  Constant3/1 -> Reshape/1
  Local Wheel Layout/1 -> Local Wheel Positions/1
  Selector3/1 -> Mux3/1
  WheelsValid/1 -> CalcAverageValidHeights/2(Valid)
  WheelHeights/1 -> CalcAverageValidHeights/1(Height)
  Mux2/1 -> WheelAngVel/1
  Speed to Front Ang Vel/1 -> Mux2/1, Mux2/2
  Bias1/1 -> Switch5/3
  Initial Ori/1 -> Selector1/1, Selector/1
  Selector1/1 -> Trigonometric Function/1
  Selector/1 -> Trigonometric Function/2
  Build Orientaion Matrix/1 -> Forward Vector/1, [LocalOri], Orientation/1
  Constant1/1 -> Build Orientaion Matrix/3
  Constant/1 -> Build Orientaion Matrix/2
  Heading/1 -> MATLAB Function1/2(currentOrientation), Build Orientaion Matrix/1
  Min Width Pulse/1 -> Switch/2
  Selector2/1 -> Bias1/1
  Reset2/1 -> Min Width Pulse/1
  Switch/1 -> [LocalPos], Position/1, MATLAB Function1/1(currentPosition)
  CoG Height/1 -> Mux3/2
  Mux3/1 -> Switch/3
  Forward Vector/1 -> Product/1, Product1/2
  Initial Pos/1 -> Position Integrator/3
  Reset/1 -> Heading/2
  Reset1/1 -> Position Integrator/2
  Trigonometric Function/1 -> Heading/3
  Yaw Rate Dead Zone/1(Yaw Rate) -> Heading/1
  CalcAverageValidHeights/1(AvHeight) -> CoG Height/1
  Product/1 -> Velocity/1, Position Integrator/1
  Brake/1 -> Gain/1
  Position Integrator/1 -> Selector2/1, Switch/1, Selector3/1
  Speed/1 -> Yaw Rate Dead Zone/2(Vel), Product/2, Speed to Rear Ang Vel/1, Speed to Front Ang Vel/1, Square/1
  g/1 -> [LocalAccel], Minus/1
  Gain/1 -> Subtract/2
  Constant2/1 -> g/1, Throttle_PID/1
  MATLAB Function/1(lateralError) -> PID Controller1/1, latError/1

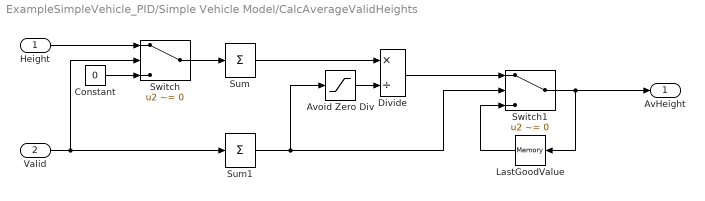
== system ExampleSimpleVehicle_PID/Simple Vehicle Model/CalcAverageValidHeights ==
  Height : Inport
  Valid : Inport  Port=2
  Avoid Zero Div : Saturate  UpperLimit=10  LowerLimit=1
  Constant : Constant  Value=0
  Divide : Product  Inputs=*/
  LastGoodValue : Memory
  Sum : Sum  Inputs=+
  Sum1 : Sum  Inputs=+
  Switch : Switch  Criteria=u2 ~= 0  SaturateOnIntegerOverflow=off  InputSameDT=off
  Switch1 : Switch  Criteria=u2 ~= 0  SaturateOnIntegerOverflow=off  InputSameDT=off
  AvHeight : Outport  VectorParamsAs1DForOutWhenUnconnected=off
  wires:
  LastGoodValue/1 -> Switch1/3
  Switch1/1 -> LastGoodValue/1, AvHeight/1
  Divide/1 -> Switch1/1
  Height/1 -> Switch/1
  Sum1/1 -> Avoid Zero Div/1, Switch1/2
  Sum/1 -> Divide/1
  Constant/1 -> Switch/3
  Valid/1 -> Switch/2, Sum1/1
  Avoid Zero Div/1 -> Divide/2
  Switch/1 -> Sum/1

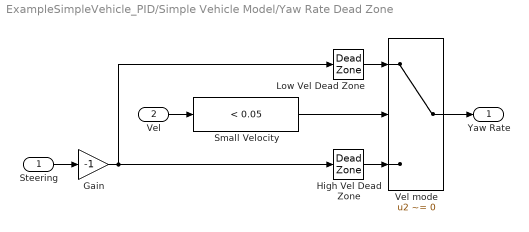
== system ExampleSimpleVehicle_PID/Simple Vehicle Model/Yaw Rate Dead Zone ==
  Steering : Inport
  Vel : Inport  Port=2
  Gain : Gain  Gain=-1
  High Vel Dead Zone : DeadZone  LowerValue=-0.01  UpperValue=0.01
  Low Vel Dead Zone : DeadZone  LowerValue=-0.02  UpperValue=0.02
  Small Velocity : simulink/Logic and Bit Operations/Compare To Constant  relop=<  const=0.05  OutDataTypeStr=boolean
  Vel mode : Switch  Criteria=u2 ~= 0  SaturateOnIntegerOverflow=off  InputSameDT=off
  Yaw Rate : Outport  VectorParamsAs1DForOutWhenUnconnected=off
  wires:
  Small Velocity/1 -> Vel mode/2
  Gain/1 -> High Vel Dead Zone/1, Low Vel Dead Zone/1
  High Vel Dead Zone/1 -> Vel mode/3
  Low Vel Dead Zone/1 -> Vel mode/1
  Vel/1 -> Small Velocity/1
  Steering/1 -> Gain/1
  Vel mode/1 -> Yaw Rate/1

== matlab function ExampleSimpleVehicle_PID/Simple Vehicle Model/MATLAB Function1 ==
  data: currentPosition input; CTE output; currentOrientation input
function CTE  = calculateCTE(currentPosition, currentOrientation)

    % AIW_data = readtable("path_with_target_speeds.csv");
    % 
    % AIW_data = load('AIW_data.mat');
    % AIW_data = AIW_data.AIW_data;

    xRef = [-293.551;-288.888;-284.234;-279.706;-275.116;-270.658;-266.15;-261.572;-257.07;-252.512;-248.118;-243.621;-238.948;-234.252;-229.748;-225.108;-220.448;-215.821;-211.368;-206.689;-202.019;-197.514;-192.734;-188.173;-183.409;-178.862;-174.111;-169.518;-165.028;-160.426;-155.615;-150.805;-145.972;-141.051;-136.113;-131.172;-126.225;-121.479;-116.839;-112.231;-107.63;-103.293;-99.172;-95.29000000000001;-91.904;-88.824;-86.108;-83.89400000000001;-82.10899999999999;-80.684;-79.68300000000001;-79.193;-79.18300000000001;-79.658;-80.649;-82.20099999999999;-84.31699999999999;-86.785;-89.604;-92.767;-96.381;-100.164;-103.811;-107.724;-111.675;-115.986;-120.236;-124.445;-128.896;-133.178;-137.479;-142.074;-146.662;-151.29;-155.903;-160.379;-165.098;-169.788;-174.364;-179.038;-183.745;-188.228;-192.718;-197.269;-202.011;-206.683;-211.409;-216.257;-221.024;-225.706;-230.57;-235.133;-239.716;-244.441;-249.136;-254.059;-258.81;-263.396;-267.885;-272.623;-277.325;-282.002;-286.667;-291.335;-296.087;-300.986;-305.893;-310.844;-315.998;-321.066;-326.146;-330.974;-335.709;-340.226;-344.401;-348.189;-351.562;-354.727;-357.385;-359.545;-361.269;-362.446;-363.009;-362.989;-362.43;-361.461;-360.141;-358.422;-356.517;-354.364;-351.832;-348.878;-345.485;-341.805;-337.808;-333.74;-329.372;-324.962;-320.24;-315.421;-310.547;-305.622;-300.983;-295.871;-293.551];
    yRef = [120.76;118.825;116.842;114.853;112.781;110.706;108.557;106.337;104.119;101.864;99.68000000000001;97.468;95.202;92.95399999999999;90.816;88.64100000000001;86.476;84.33799999999999;82.28700000000001;80.133;77.992;75.929;73.742;71.66;69.489;67.423;65.215;63.032;60.983;59.012;57.162;55.579;54.254;53.207;52.477;52.114;52.128;52.535;53.339;54.576;56.315;58.48;61.098;64.18600000000001;67.51300000000001;71.221;75.244;79.294;83.43600000000001;87.85599999999999;92.52200000000001;97.104;101.631;106.185;110.719;115.231;119.589;123.497;127.058;130.363;133.534;136.478;139.166;141.952;144.692;147.648;150.455;153.125;155.837;158.328;160.715;163.155;165.494;167.811;170.108;172.314;174.579;176.754;178.835;180.936;183.034;185.024;187.019;189.059;191.192;193.299;195.435;197.628;199.787;201.908;204.114;206.183;208.261;210.4;212.524;214.752;216.904;218.983;221.024;223.267;225.473;227.568;229.528;231.326;232.933;234.293;235.281;235.855;235.952;235.548;234.588;233.119;231.095;228.573;225.646;222.369;218.821;214.936;210.919;206.774;202.29;197.492;192.641;187.711;182.837;178.179;173.61;168.926;164.401;160.123;155.893;151.763;147.807;144.2;140.924;138.089;135.47;133.183;131.051;129.127;127.306;125.535;123.749;121.711;120.76];
    vRef = [70;66.2941526152573;65.4883647028928;66.0806810173367;65.26896339678061;66.38411146223039;67.3958387030261;67.44592545744069;69.329950287306;69.1882758068728;68.3399139325445;67.8708656511444;68.0298306929415;68.5896149793253;68.1152248297563;68.63555972456859;69.1481986236618;69.4599993837293;69.9252960878933;69.3639988911179;69.8107068477354;69.8743668318338;69.619725001083;69.7562053585058;69.5126574618636;66.8719643020907;66.5091815156028;63.7827888901593;61.4788133988011;57.7449016550197;53.9974942907394;53.6605244902812;52.084372378414;50.7040292465574;48.3551543600423;47.8757137938598;45.44230021571;45.0547902412987;44.8125277874768;44.1542423154531;42.7562947109367;43.0237595384218;42.9484526008551;41.4257959721631;43.2571984505023;43.5174230788054;42.7218682523597;42.8210740638573;43.8798605976025;43.3680625384228;41.050532484812;41.1167068038216;41.5115895718732;40.9821406887103;40.9724706479303;40.3572685751828;39.8779433001052;40.8523153006594;43.4782648280148;46.1514165633422;51.1173397417285;59.1586834051362;63.8222944745662;64.9860662503273;68.09774394366831;63.3540045110797;62.8833170176386;63.6684950949253;61.9666887077676;62.2677836847414;63.582020518799;63.7412538286618;67.1728885787014;69.1240638051038;68.2678328545159;66.2320071591884;64.9379557107406;66.9499315721812;68.288600479504;68.7439476332636;69.3231332765677;69.8500899327105;68.66563066099511;69.50160418981601;69.596479219993;69.6746981329475;69.8776836020929;69.8129239020713;69.9633846068996;69.8356926516352;69.9605815921807;69.99484195273639;69.76728865106691;69.8972515280409;69.946697957835;69.8660412195262;69.8644375826603;69.5234982627379;64.634943151824;68.6108023038381;63.4034940082739;61.3828028681508;59.1949084097623;56.0993056497234;52.9563000761606;48.6600632149421;46.5811102623243;45.3740766116321;44.0924658888451;43.4590924152461;42.1678712337758;43.2439583256756;43.5724926564217;43.4993836022364;43.2285780638725;43.4716042905227;48.3773165515135;42.6594142234564;41.4769704966752;41.490023311183;40.1153820764336;39.439060283349;40.7167392521961;41.7807093964386;44.0168794632518;47.2964084120581;49.8703327366803;54.2578101978239;48.7811919622444;48.888182493106;47.7142112915798;46.8807887059169;46.4014281715362;46.2575661895888;46.9478486843666;50.2626308688873;50.659172156746;53.7892565325441;55.7629716999758;62.0428321692388;65.39425033502739;61.3094080047088;66.1398697765437;55.8306766985528;70];

    AIW_data = [xRef, yRef, vRef];
    xV = currentPosition(1);
    yV = currentPosition(2);

    % Find nearest AIW waypoint using Euclidean distance
    d = sqrt((AIW_data(:,1) - xV).^2 + (AIW_data(:,2) -yV).^2);
    [minDist, closestWaypointIdx] = min(d);

    closestWaypoint = [AIW_data(closestWaypointIdx, 1), AIW_data(closestWaypointIdx, 2)];
    xI = AIW_data(closestWaypointIdx, 1);
    yI = AIW_data(closestWaypointIdx, 2);

    if closestWaypointIdx ~= size(AIW_data, 1)
        xI_1 = AIW_data(closestWaypointIdx+1, 1);
        yI_1 = AIW_data(closestWaypointIdx+1, 2);
    else
        xI_1 = AIW_data(1, 1);
        yI_1 = AIW_data(1, 2);
    end

    % Segment between path points
    p = [xI_1 - xI; yI_1 - yI];

    % Vector from path to vehicle
    v = [xV - xI; yV - yI];

    % Projection of v onto p
    dotP = dot(p, v);
    pMagSquared = dot(p, p);
    proj_v_on_p = (dotP / pMagSquared) * p;

    % Calc residual vect
    residual = v - proj_v_on_p;

    % CTE
    CTE = norm(residual);

    % Get the sign of CTE
    crossProd = p(1) * v(2) - p(2) * v(1);
    if crossProd > 0

        CTE = CTE; % Left of path

    else

        CTE = -CTE; % Right of path

    end



    % Fetch ref vel
    refVel = AIW_data(closestWaypointIdx, 3);


end

== matlab function ExampleSimpleVehicle_PID/Simple Vehicle Model/MATLAB Function ==
  data: currentPosition input; lateralError output; refVel output
function [lateralError, refVel] = calculateLateralError(currentPosition)

    % AIW_data = readtable("path_with_target_speeds.csv");
    % 
    % AIW_data = load('AIW_data.mat');
    % AIW_data = AIW_data.AIW_data;

    xRef = [-293.551;-288.888;-284.234;-279.706;-275.116;-270.658;-266.15;-261.572;-257.07;-252.512;-248.118;-243.621;-238.948;-234.252;-229.748;-225.108;-220.448;-215.821;-211.368;-206.689;-202.019;-197.514;-192.734;-188.173;-183.409;-178.862;-174.111;-169.518;-165.028;-160.426;-155.615;-150.805;-145.972;-141.051;-136.113;-131.172;-126.225;-121.479;-116.839;-112.231;-107.63;-103.293;-99.172;-95.29000000000001;-91.904;-88.824;-86.108;-83.89400000000001;-82.10899999999999;-80.684;-79.68300000000001;-79.193;-79.18300000000001;-79.658;-80.649;-82.20099999999999;-84.31699999999999;-86.785;-89.604;-92.767;-96.381;-100.164;-103.811;-107.724;-111.675;-115.986;-120.236;-124.445;-128.896;-133.178;-137.479;-142.074;-146.662;-151.29;-155.903;-160.379;-165.098;-169.788;-174.364;-179.038;-183.745;-188.228;-192.718;-197.269;-202.011;-206.683;-211.409;-216.257;-221.024;-225.706;-230.57;-235.133;-239.716;-244.441;-249.136;-254.059;-258.81;-263.396;-267.885;-272.623;-277.325;-282.002;-286.667;-291.335;-296.087;-300.986;-305.893;-310.844;-315.998;-321.066;-326.146;-330.974;-335.709;-340.226;-344.401;-348.189;-351.562;-354.727;-357.385;-359.545;-361.269;-362.446;-363.009;-362.989;-362.43;-361.461;-360.141;-358.422;-356.517;-354.364;-351.832;-348.878;-345.485;-341.805;-337.808;-333.74;-329.372;-324.962;-320.24;-315.421;-310.547;-305.622;-300.983;-295.871;-293.551];
    yRef = [120.76;118.825;116.842;114.853;112.781;110.706;108.557;106.337;104.119;101.864;99.68000000000001;97.468;95.202;92.95399999999999;90.816;88.64100000000001;86.476;84.33799999999999;82.28700000000001;80.133;77.992;75.929;73.742;71.66;69.489;67.423;65.215;63.032;60.983;59.012;57.162;55.579;54.254;53.207;52.477;52.114;52.128;52.535;53.339;54.576;56.315;58.48;61.098;64.18600000000001;67.51300000000001;71.221;75.244;79.294;83.43600000000001;87.85599999999999;92.52200000000001;97.104;101.631;106.185;110.719;115.231;119.589;123.497;127.058;130.363;133.534;136.478;139.166;141.952;144.692;147.648;150.455;153.125;155.837;158.328;160.715;163.155;165.494;167.811;170.108;172.314;174.579;176.754;178.835;180.936;183.034;185.024;187.019;189.059;191.192;193.299;195.435;197.628;199.787;201.908;204.114;206.183;208.261;210.4;212.524;214.752;216.904;218.983;221.024;223.267;225.473;227.568;229.528;231.326;232.933;234.293;235.281;235.855;235.952;235.548;234.588;233.119;231.095;228.573;225.646;222.369;218.821;214.936;210.919;206.774;202.29;197.492;192.641;187.711;182.837;178.179;173.61;168.926;164.401;160.123;155.893;151.763;147.807;144.2;140.924;138.089;135.47;133.183;131.051;129.127;127.306;125.535;123.749;121.711;120.76];
    vRef = [70;66.2941526152573;65.4883647028928;66.0806810173367;65.26896339678061;66.38411146223039;67.3958387030261;67.44592545744069;69.329950287306;69.1882758068728;68.3399139325445;67.8708656511444;68.0298306929415;68.5896149793253;68.1152248297563;68.63555972456859;69.1481986236618;69.4599993837293;69.9252960878933;69.3639988911179;69.8107068477354;69.8743668318338;69.619725001083;69.7562053585058;69.5126574618636;66.8719643020907;66.5091815156028;63.7827888901593;61.4788133988011;57.7449016550197;53.9974942907394;53.6605244902812;52.084372378414;50.7040292465574;48.3551543600423;47.8757137938598;45.44230021571;45.0547902412987;44.8125277874768;44.1542423154531;42.7562947109367;43.0237595384218;42.9484526008551;41.4257959721631;43.2571984505023;43.5174230788054;42.7218682523597;42.8210740638573;43.8798605976025;43.3680625384228;41.050532484812;41.1167068038216;41.5115895718732;40.9821406887103;40.9724706479303;40.3572685751828;39.8779433001052;40.8523153006594;43.4782648280148;46.1514165633422;51.1173397417285;59.1586834051362;63.8222944745662;64.9860662503273;68.09774394366831;63.3540045110797;62.8833170176386;63.6684950949253;61.9666887077676;62.2677836847414;63.582020518799;63.7412538286618;67.1728885787014;69.1240638051038;68.2678328545159;66.2320071591884;64.9379557107406;66.9499315721812;68.288600479504;68.7439476332636;69.3231332765677;69.8500899327105;68.66563066099511;69.50160418981601;69.596479219993;69.6746981329475;69.8776836020929;69.8129239020713;69.9633846068996;69.8356926516352;69.9605815921807;69.99484195273639;69.76728865106691;69.8972515280409;69.946697957835;69.8660412195262;69.8644375826603;69.5234982627379;64.634943151824;68.6108023038381;63.4034940082739;61.3828028681508;59.1949084097623;56.0993056497234;52.9563000761606;48.6600632149421;46.5811102623243;45.3740766116321;44.0924658888451;43.4590924152461;42.1678712337758;43.2439583256756;43.5724926564217;43.4993836022364;43.2285780638725;43.4716042905227;48.3773165515135;42.6594142234564;41.4769704966752;41.490023311183;40.1153820764336;39.439060283349;40.7167392521961;41.7807093964386;44.0168794632518;47.2964084120581;49.8703327366803;54.2578101978239;48.7811919622444;48.888182493106;47.7142112915798;46.8807887059169;46.4014281715362;46.2575661895888;46.9478486843666;50.2626308688873;50.659172156746;53.7892565325441;55.7629716999758;62.0428321692388;65.39425033502739;61.3094080047088;66.1398697765437;55.8306766985528;70];

    AIW_data = [xRef, yRef, vRef];
    x = currentPosition(1);
    y = currentPosition(2);
    currentPoint = [x, y];

    % Find nearest AIW waypoint using Euclidean distance
    d = sqrt((AIW_data(:,1) - x).^2 + (AIW_data(:,2) -y).^2);
    [minDist, closestWaypointIdx] = min(d);

    closestWaypoint = [AIW_data(closestWaypointIdx, 1), AIW_data(closestWaypointIdx, 2)];

    dx = closestWaypoint(1) - x;
    dy = closestWaypoint(2) - y;

    % Path angle at the closest point
    pathAngle = atan2(dy, dx);

    % Calculate error between heading and path angle
    errorAngle = pathAngle - currentOrientation(1);
    lateralError = minDist * sin(errorAngle); 


    % Fetch ref vel
    refVel = AIW_data(closestWaypointIdx, 3);


end
